simulink model "motes"  (Simulink 4.00)
settings: Solver=ode45  StartTime=0.0  StopTime=40  RelTol=1e-3
PostLoadFcn:
  | init
InitFcn:
  | clear functions
values from neighbouring files (symbols this model uses):
  nbrOfMotes = 3    [init.m]
  xPos = [-18 -18 -18]    [init.m]
  yPos = [-18 -18 -18]    [init.m]
undefined symbols (not defined in the file or in its folder): WLAN
libraries: truetime x3
settings Model: Creator=mandersson  LastModifiedBy=anton  SaveTime=off  SaveOutput=off  RTWOptions="-aEnforceIntegerDowncast=1 -aExtMode=0 -aFoldNonRolledExpr=1 -aForceParamTrailComments=0 -aGenerateComments=1 -aIgnoreCustomStorageClasses=0 -aIncHierarchyInIds=0 -aInlineInvariantSignals=0 -aLocalBlockOutputs=1 -aLogVarNameModifier=\"rt_\" -aRTWVerbose=1 -aRollThreshold=5 -aShowEliminatedStatements=0"  ExtModeAutoUpdateStatusClock=off  BooleanDataType=on

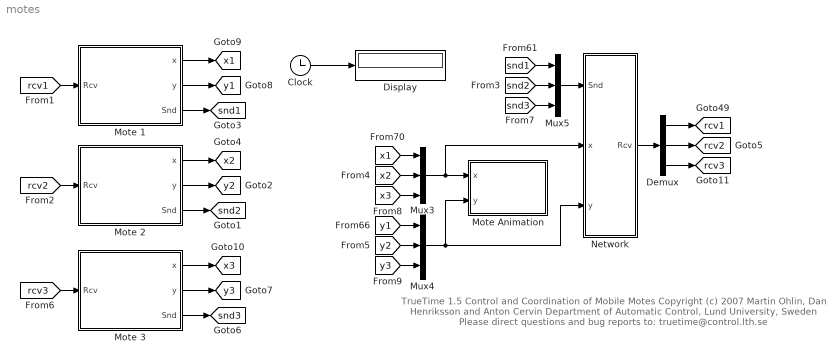
== system motes ==
  note: TrueTime 1.5  Control and Coordination of Mobile Motes
      | Copyright (c) 2007
      | Martin Ohlin, Dan Henriksson and Anton Cervin
      | Department of Automatic Control, Lund University, Sweden
      | Please direct questions and bug reports to:  truetime@control.lth.se
  Clock : Clock
      settings: DisplayTime=off  Decimation=10
  Demux : Demux  Outputs=nbrOfMotes  BusSelectionMode=off
  Display : Display
      settings: Format=short
  Mote 1 : Subsystem  mask(MOTE){x0=xPos(1), y0=yPos(1)}
      settings: RTWFcnNameOpts=Auto  RTWFileNameOpts=Auto
  Mote 2 : Subsystem  mask(MOTE){x0=xPos(2), y0=yPos(2)}
      settings: RTWFcnNameOpts=Auto  RTWFileNameOpts=Auto
  Mote 3 : Subsystem  mask(MOTE){x0=xPos(3), y0=yPos(3)}
      settings: RTWFcnNameOpts=Auto  RTWFileNameOpts=Auto
  Mote Animation : Subsystem  mask{numMotes=nbrOfMotes, xmax=20, ymax=20, ts=0.1, x0=xPos, y0=yPos}
      mask prompts: numMotes "Number of Motes"; ts "Update period"
      settings: RTWFcnNameOpts=Auto  RTWFileNameOpts=Auto
  Mux3 : Mux  Inputs=nbrOfMotes
  Mux4 : Mux  Inputs=nbrOfMotes
  Mux5 : Mux  Inputs=nbrOfMotes
  Network : Subsystem
      settings: RTWFcnNameOpts=Auto  RTWFileNameOpts=Auto
  tag scope: rcv1=global, rcv2=global, rcv3=global, snd1=global, snd2=global, snd3=global, x1=global, x2=global, x3=global, y1=global, y2=global, y3=global
  wires:
  Mote 1/1(x) -> [x1]
  Mote 1/2(y) -> [y1]
  [rcv1] -> Mote 1/1(Rcv)
  Mote 1/3(Snd) -> [snd1]
  Mux3/1 -> Mote Animation/1(x), Network/2(x)
  Mux4/1 -> Mote Animation/2(y), Network/3(y)
  Network/1(Rcv) -> Demux/1
  Mux5/1 -> Network/1(Snd)
  Demux/1 -> [rcv1]
  Clock/1 -> Display/1
  Mote 2/1(x) -> [x2]
  Mote 2/2(y) -> [y2]
  [rcv2] -> Mote 2/1(Rcv)
  Mote 2/3(Snd) -> [snd2]
  Demux/2 -> [rcv2]
  Mote 3/1(x) -> [x3]
  Mote 3/2(y) -> [y3]
  [rcv3] -> Mote 3/1(Rcv)
  Mote 3/3(Snd) -> [snd3]
  Demux/3 -> [rcv3]
  [snd1] -> Mux5/1
  [snd2] -> Mux5/2
  [snd3] -> Mux5/3
  [x1] -> Mux3/1
  [x2] -> Mux3/2
  [x3] -> Mux3/3
  [y1] -> Mux4/1
  [y2] -> Mux4/2
  [y3] -> Mux4/3

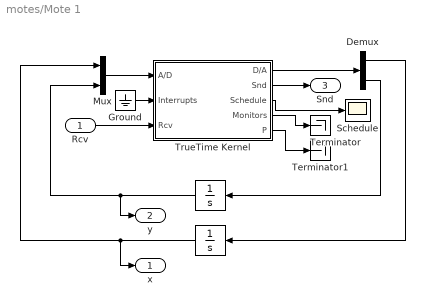
== system motes/Mote 1 ==
  Rcv : Inport  Port=1  LatchInput=off
  " " : Integrator  Orientation=left  ExternalReset=none  InitialConditionSource=internal  InitialCondition=y0  LimitOutput=off  UpperSaturationLimit=inf  LowerSaturationLimit=-inf  ShowSaturationPort=off  ShowStatePort=off  AbsoluteTolerance=auto
  "    " : Integrator  Orientation=left  ExternalReset=none  InitialConditionSource=internal  InitialCondition=x0  LimitOutput=off  UpperSaturationLimit=inf  LowerSaturationLimit=-inf  ShowSaturationPort=off  ShowStatePort=off  AbsoluteTolerance=auto
  Demux : Demux  Outputs=2  BusSelectionMode=off
  Ground : Ground
  Mux : Mux  Inputs=2
  Schedule : Scope
      settings: TickLabels=on  TimeRange=3.5  YMin=1.8  YMax=3.7  SaveToWorkspace=off  SaveName=ScopeData  DataFormat=Array  MaxDataPoints=5000
  Terminator : Terminator
  Terminator1 : Terminator
  TrueTime Kernel : Subsystem  AncestorBlock=truetime/TrueTime Kernel  mask{sfun=node_init, args=1, battery=off, clockdrift=0, clockoffset=0}
      mask prompts: sfun "Name of init function (MEX or MATLAB)"; args "Init function argument"; clockdrift "Clock drift"; clockoffset "Clock offset"
      settings: RTWFcnNameOpts=Auto  RTWFileNameOpts=Auto
      mask CallbackString: ||batterychange||
  x : Outport  Port=1
  y : Outport  Port=2
  Snd : Outport  Port=3
  wires:
  "    "/1 -> x/1, Mux/1
  " "/1 -> y/1, Mux/2
  Demux/1 -> "    "/1
  Demux/2 -> " "/1
  TrueTime Kernel/2(Snd) -> Snd/1
  TrueTime Kernel/1(D/A) -> Demux/1
  TrueTime Kernel/4(Monitors) -> Terminator/1
  Mux/1 -> TrueTime Kernel/1(A/D)
  Rcv/1 -> TrueTime Kernel/3(Rcv)
  Ground/1 -> TrueTime Kernel/2(Interrupts)
  TrueTime Kernel/3(Schedule) -> Schedule/1
  TrueTime Kernel/5(P) -> Terminator1/1

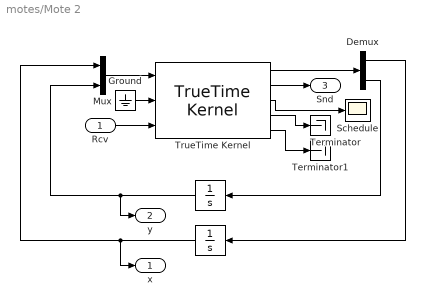
== system motes/Mote 2 ==
  Rcv : Inport  Port=1  LatchInput=off
  " " : Integrator  Orientation=left  ExternalReset=none  InitialConditionSource=internal  InitialCondition=y0  LimitOutput=off  UpperSaturationLimit=inf  LowerSaturationLimit=-inf  ShowSaturationPort=off  ShowStatePort=off  AbsoluteTolerance=auto
  "    " : Integrator  Orientation=left  ExternalReset=none  InitialConditionSource=internal  InitialCondition=x0  LimitOutput=off  UpperSaturationLimit=inf  LowerSaturationLimit=-inf  ShowSaturationPort=off  ShowStatePort=off  AbsoluteTolerance=auto
  Demux : Demux  Outputs=2  BusSelectionMode=off
  Ground : Ground
  Mux : Mux  Inputs=2
  Schedule : Scope
      settings: TickLabels=on  TimeRange=3.5  YMin=1.8  YMax=3.7  SaveToWorkspace=off  SaveName=ScopeData  DataFormat=Array  MaxDataPoints=5000
  Terminator : Terminator
  Terminator1 : Terminator
  TrueTime Kernel : truetime/TrueTime Kernel  sfun=node_init  args=2  battery=off  clockdrift=0  clockoffset=0
  x : Outport  Port=1
  y : Outport  Port=2
  Snd : Outport  Port=3
  wires:
  "    "/1 -> x/1, Mux/1
  " "/1 -> y/1, Mux/2
  Demux/1 -> "    "/1
  Demux/2 -> " "/1
  TrueTime Kernel/2 -> Snd/1
  TrueTime Kernel/1 -> Demux/1
  TrueTime Kernel/4 -> Terminator/1
  Mux/1 -> TrueTime Kernel/1
  Rcv/1 -> TrueTime Kernel/3
  Ground/1 -> TrueTime Kernel/2
  TrueTime Kernel/3 -> Schedule/1
  TrueTime Kernel/5 -> Terminator1/1

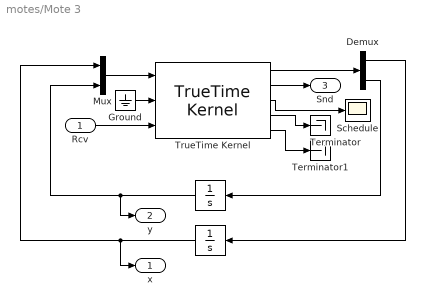
== system motes/Mote 3 ==
  Rcv : Inport  Port=1  LatchInput=off
  " " : Integrator  Orientation=left  ExternalReset=none  InitialConditionSource=internal  InitialCondition=y0  LimitOutput=off  UpperSaturationLimit=inf  LowerSaturationLimit=-inf  ShowSaturationPort=off  ShowStatePort=off  AbsoluteTolerance=auto
  "    " : Integrator  Orientation=left  ExternalReset=none  InitialConditionSource=internal  InitialCondition=x0  LimitOutput=off  UpperSaturationLimit=inf  LowerSaturationLimit=-inf  ShowSaturationPort=off  ShowStatePort=off  AbsoluteTolerance=auto
  Demux : Demux  Outputs=2  BusSelectionMode=off
  Ground : Ground
  Mux : Mux  Inputs=2
  Schedule : Scope
      settings: TickLabels=on  TimeRange=3.5  YMin=1.8  YMax=3.7  SaveToWorkspace=off  SaveName=ScopeData  DataFormat=Array  MaxDataPoints=5000
  Terminator : Terminator
  Terminator1 : Terminator
  TrueTime Kernel : truetime/TrueTime Kernel  sfun=node_init  args=3  battery=off  clockdrift=0  clockoffset=0
  x : Outport  Port=1
  y : Outport  Port=2
  Snd : Outport  Port=3
  wires:
  "    "/1 -> x/1, Mux/1
  " "/1 -> y/1, Mux/2
  Demux/1 -> "    "/1
  Demux/2 -> " "/1
  TrueTime Kernel/2 -> Snd/1
  TrueTime Kernel/1 -> Demux/1
  TrueTime Kernel/4 -> Terminator/1
  Mux/1 -> TrueTime Kernel/1
  Rcv/1 -> TrueTime Kernel/3
  Ground/1 -> TrueTime Kernel/2
  TrueTime Kernel/3 -> Schedule/1
  TrueTime Kernel/5 -> Terminator1/1

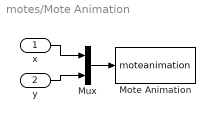
== system motes/Mote Animation ==
  x : Inport  Port=1  LatchInput=off
  y : Inport  Port=2  LatchInput=off
  Mote Animation : S-Function  FunctionName=moteanimation  Parameters=[numMotes ts xmax ymax] x0 y0  PortCounts=[]  SFunctionModules=''
      settings: DeleteFcn=if ~isempty(findobj('type','figure','name','dblpend1 Animation'));close('dblpend1 Animation'); end;
  Mux : Mux  Inputs=2
  wires:
  Mux/1 -> Mote Animation/1
  y/1 -> Mux/2
  x/1 -> Mux/1

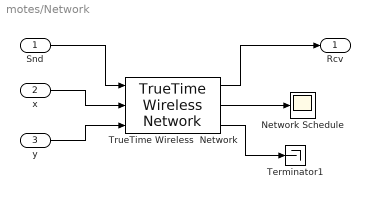
== system motes/Network ==
  Snd : Inport  Port=1  LatchInput=off
  x : Inport  Port=2  LatchInput=off
  y : Inport  Port=3  LatchInput=off
  Network Schedule : Scope
      settings: TimeRange=40  YMin=1  YMax=3.5  SaveToWorkspace=off  SaveName=nschedule  MaxDataPoints=5000
  Terminator1 : Terminator
  TrueTime Wireless  Network : truetime/TrueTime Wireless  Network  nwtype=802.11b (WLAN)  nwnbr=1  nnodes=nbrOfMotes  rate=800000  minsize=272  transpower=transmitPower  threshold=receiverThreshold  pathloss=pathloss  use_pathloss_function=off  acktimeout=0.00004  retrylimit=5  error_threshold=errorCodingThreshold
  Rcv : Outport  Port=1
  wires:
  TrueTime Wireless  Network/1 -> Rcv/1
  TrueTime Wireless  Network/2 -> Network Schedule/1
  Snd/1 -> TrueTime Wireless  Network/1
  y/1 -> TrueTime Wireless  Network/3
  x/1 -> TrueTime Wireless  Network/2
  TrueTime Wireless  Network/3 -> Terminator1/1

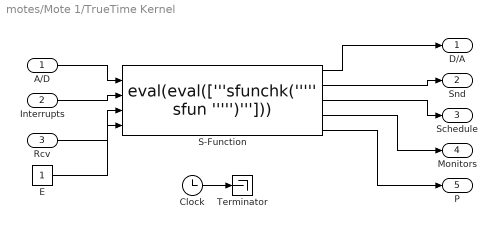
== system motes/Mote 1/TrueTime Kernel ==
  A/D : Inport  Port=1  LatchInput=off
  Interrupts : Inport  Port=2  LatchInput=off
  Rcv : Inport  Port=3  LatchInput=off
  Clock : Clock
      settings: DisplayTime=off  Decimation=10
  E : Constant  Value=1
  S-Function : S-Function  FunctionName=eval(eval(['''sfunchk(''''' sfun ''''')''']))  Parameters=sfun, args, clockdrift, clockoffset  PortCounts=[]  SFunctionModules=''
  Terminator : Terminator
  D/A : Outport  Port=1
  Snd : Outport  Port=2
  Schedule : Outport  Port=3
  Monitors : Outport  Port=4
  P : Outport  Port=5
  wires:
  Clock/1 -> Terminator/1
  Rcv/1 -> S-Function/3
  Interrupts/1 -> S-Function/2
  S-Function/4 -> Monitors/1
  S-Function/3 -> Schedule/1
  S-Function/1 -> D/A/1
  S-Function/2 -> Snd/1
  A/D/1 -> S-Function/1
  E/1 -> S-Function/4
  S-Function/5 -> P/1
